simulink model "sfit_test"  (R2017a)
settings: Solver=VariableStepAuto  StartTime=0.0  StopTime=10.0  RelTol=1e-3
settings Model: Creator=Devansh  LastModifiedBy=Devansh

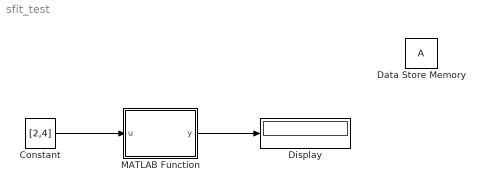
== system sfit_test ==
  Constant : Constant  Value=[2,4]
  Data Store Memory : DataStoreMemory  ReadBeforeWriteMsg=warning  WriteAfterWriteMsg=warning  WriteAfterReadMsg=warning  ShowAdditionalParam=off
  Display : Display
      settings: Decimation=2
  MATLAB Function : MATLAB Function  TreatAsAtomicUnit=on
  wires:
  MATLAB Function/1(y) -> Display/1
  Constant/1 -> MATLAB Function/1(u)

== matlab function sfit_test/MATLAB Function ==
  data: u input; y output
function y = fcn(u)

c=load('./SSTOL_Aero_Model/cl_fit40.mat');

y = c.cl_fit_40(u(1),u(2));
